simulink model "sampleModel1710"  (R2023a)
settings: Solver=VariableStepAuto  StartTime=0.0  StopTime=10.0  RelTol=1e-3
libraries: hdlsllib x4, simulink x3
settings Model: Creator=user1  LastModifiedBy=user1

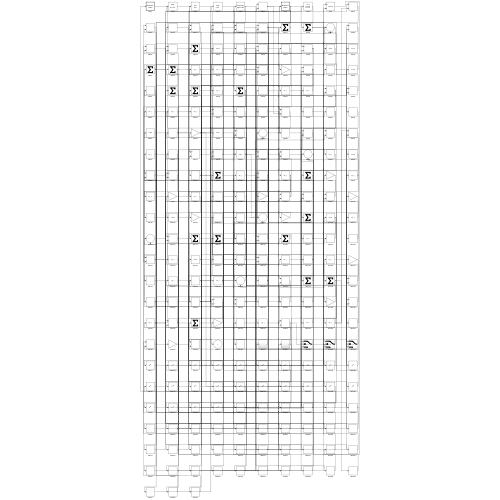
[thumbnail: Simulink's stored preview of the top-level diagram]
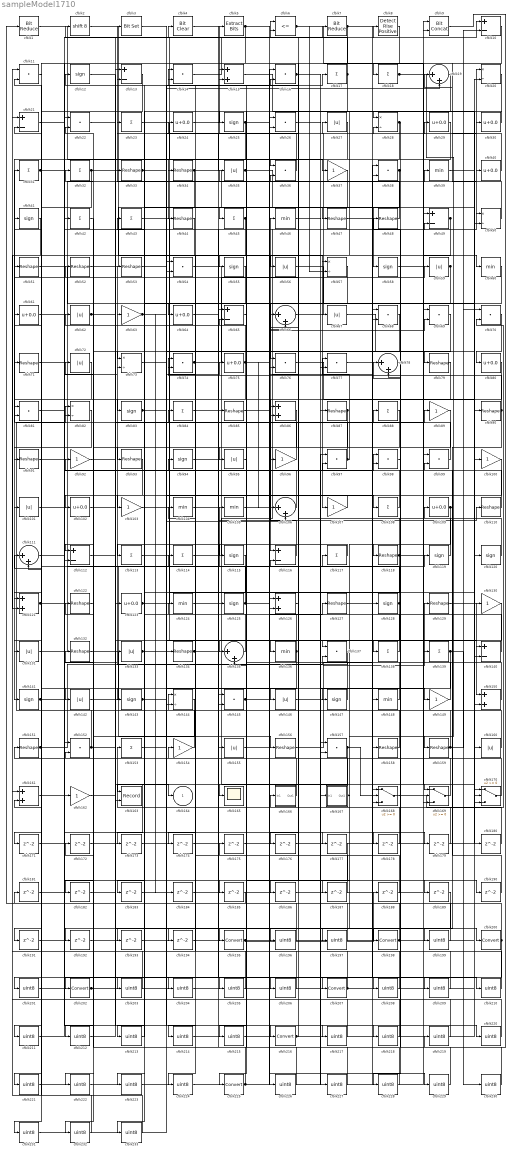
== system sampleModel1710 ==
  cfblk1 : hdlsllib/Logic and Bit Operations/Bit Reduce  mode=AND
  cfblk{10,13,21,49,65,112,116,140} (8 alike) : Sum  Inputs=+-
  cfblk{37,63,89,92,96,100,103,107,130,149,154,162} (12 alike) : Gain
  cfblk{27,35,56,59,62,67,72,95,101,131,133,142,146,155,160} (15 alike) : Abs  SaturateOnIntegerOverflow=off
  cfblk{24,29..30,40,61,64,75,80,102,109,123} (11 alike) : Bias  Bias=0.0  SaturateOnIntegerOverflow=off
  cfblk{39,46,60,104..105,124,136,148} (8 alike) : MinMax
  cfblk{19,66,78,106,111,135} (6 alike) : Sum  Inputs=|++
  cfblk{17..18,23,31..32,42..43,45,84,88,108,113..114,117,138..139,153} (17 alike) : Sum  Inputs=+
  cfblk{11,14,16,22,26,36,38,54,68..70,74,76..77,81,97..99,137,145,152,157} (22 alike) : DotProduct  OutDataTypeStr=Inherit: Inherit via internal rule
  cfblk{33..34,44,47..48,51..53,71,79,85,87,90..91,93,110,118,122,127,129,132,134,151,156,158..159} (26 alike) : Reshape
  cfblk{12,25,41,55,58,83,94,115,119..120,125,128,141,143,147} (15 alike) : Signum
  cfblk{15,86,121,126,150,161} (6 alike) : Sum
  cfblk{20,28,50,57,73,82,144} (7 alike) : Product  Inputs=*/  RndMeth=Zero  SaturateOnIntegerOverflow=on
  cfblk163 : Record  FileSettingsInternal="{\"entries\":[{\"content\":{\"excelSettings\":{\"content\":{},\"type\":\"Streamout.ExcelSettings\"}},\"type\":\"Streamout.FileSettingStorage\",\"uuid\":\"\"}],\"packageUris\":[\"http:\\/\\/schema.mathworks.com\\/mf0\\/streamout_blocks\\/R2020a\"],\"version\":\"1.0\"}"  Layout=[1 1]  SignalsInternal="{\"entries\":[{\"content\":{\"signals\":[{\"content\":{\"blockPath\":[],\"dimensions\":[1],\"domain\":\"\",\"lineColor\":\"#a2142f\",\"plots\":[1],\"port\":1,\"signalID\":3197,\"signalName\":\"XY Graph:1\"},\"type\":\"RecordBlkView.Signal\",\"uuid\":\"\"},{\"content\":{\"blockPath\":[],\"dimensions\":[1],\"domain\":\"\",\"lineColor\":\"#139fff\",\"plots\":[1],\"port\":2,\"signalID\":3200,\"signalName\":\"XY Graph:2\"},\"type\":\"RecordBlkView.Signal\",\"uuid\":\"\"}]},\"type\":\"RecordBlkView.InputSignals\",\"uuid\":\"\"}],\"packageUris\":[\"http:\\/\\/schema.mathworks.com\\/mf0\\/streamout_blocks\\/R2020a\"],\"version\":\"1.0\"}"  VisualizationBindings="{\"xyplotplugin\":{\"info\":[{\"series\":[{\"bindingParametersList\":[{\"parameter\":\"X-Axis\",\"signalID\":3197,\"signalName\":\"XY Graph:1\"},{\"parameter\":\"Y-Axis\",\"signalID\":3200,\"signalName\":\"XY Graph:2\"}],\"seriesID\":41778}],\"subplotID\":1}]}}"  CompatibilityTag=XY  st=-1
  cfblk165 : Scope
  cfblk166 : Subsystem
      settings: LibrarySourceBlock=|
      | hdlsllib/Ports &
      | Subsystems/Subsystem
  cfblk167 : Subsystem
      settings: LibrarySourceBlock=|
      | hdlsllib/Ports &
      | Subsystems/Subsystem
  cfblk168 : Switch  SaturateOnIntegerOverflow=off  InputSameDT=off
  cfblk169 : Switch  SaturateOnIntegerOverflow=off  InputSameDT=off
  cfblk170 : Switch  SaturateOnIntegerOverflow=off  InputSameDT=off
  cfblk{171..194} (24 alike) : Delay  SampleTime=1
  cfblk{195,198,200,202,207,216,225} (7 alike) : DataTypeConversion  SaturateOnIntegerOverflow=off  RndMeth=Floor
  cfblk{196..197,199,201,203..206,208..215,217..224,226..233} (32 alike) : DataTypeConversion  OutDataTypeStr=uint8  SaturateOnIntegerOverflow=off  RndMeth=Floor
  cfblk2 : ArithShift  BitShiftNumber=8
  cfblk3 : simulink/Logic and Bit Operations/Bit Set  iBit=0
      settings: LibrarySourceBlock=|
      | hdlsllib/Logic and Bit
      | Operations/Bit Set
  cfblk4 : simulink/Logic and Bit Operations/Bit Clear  iBit=0
      settings: LibrarySourceBlock=|
      | hdlsllib/Logic and Bit
      | Operations/Bit Clear
  cfblk5 : simulink/Logic and Bit Operations/Extract Bits  bitsToExtract=Upper half  numBits=8  bitIdxRange=[0 7]  outScalingMode=Preserve fixed-point scaling
      settings: LibrarySourceBlock=|
      | hdlsllib/Logic and Bit
      | Operations/Extract Bits
  cfblk6 : RelationalOperator  Operator=<=  OutDataTypeStr=boolean  InputSameDT=off
  cfblk7 : hdlsllib/Logic and Bit Operations/Bit Reduce  mode=AND
  cfblk8 : hdlsllib/Logic and Bit Operations/Detect Rise Positive  vinit=0  OutDataTypeStr=boolean
  cfblk9 : hdlsllib/Logic and Bit Operations/Bit Concat  numInputs=2
  cfblk164 : Outport  VectorParamsAs1DForOutWhenUnconnected=off
  wires:
  cfblk167/1(Out1) -> cfblk154/1, cfblk187/1
  cfblk116/1 -> cfblk46/1
  cfblk131/1 -> cfblk39/1
  cfblk159/1 -> cfblk70/1, cfblk10/2, cfblk76/2
  cfblk154/1 -> cfblk82/1
  cfblk16/1 -> cfblk28/1, cfblk149/1, cfblk176/1
  cfblk82/1 -> cfblk141/1
  cfblk36/1 -> cfblk5/1
  cfblk27/1 -> cfblk101/1
  cfblk43/1 -> cfblk137/1
  cfblk52/1 -> cfblk45/1
  cfblk18/1 -> cfblk153/1, cfblk60/1
  cfblk137/1 -> cfblk53/1
  cfblk80/1 -> cfblk116/1
  cfblk72/1 -> cfblk131/1
  cfblk153/1 -> cfblk134/1
  cfblk123/1 -> cfblk8/1, cfblk33/1
  cfblk158/1 -> cfblk144/1
  cfblk44/1 -> cfblk93/1
  cfblk40/1 -> cfblk18/1
  cfblk108/1 -> cfblk63/1
  cfblk54/1 -> cfblk169/1
  cfblk97/1 -> cfblk32/1, cfblk77/1
  cfblk146/1 -> cfblk129/1
  cfblk170/1 -> cfblk72/1
  cfblk30/1 -> cfblk25/1
  cfblk151/1 -> cfblk137/2, cfblk133/1
  cfblk2/1 -> cfblk107/1
  cfblk168/1 -> cfblk70/2
  cfblk125/1 -> cfblk105/1, cfblk28/2
  cfblk141/1 -> cfblk42/1, cfblk201/1
  cfblk23/1 -> cfblk36/1
  cfblk95/1 -> cfblk165/1
  cfblk88/1 -> cfblk136/1
  cfblk105/1 -> cfblk20/1
  cfblk136/1 -> cfblk14/2, cfblk171/1
  cfblk50/1 -> cfblk19/1
  cfblk66/1 -> cfblk30/1
  cfblk75/1 -> cfblk62/1, cfblk82/2, cfblk106/1, cfblk69/2
  cfblk24/1 -> cfblk67/1
  cfblk74/1 -> cfblk59/1, cfblk14/1
  cfblk51/1 -> cfblk76/1
  cfblk99/1 -> cfblk31/1
  cfblk65/1 -> cfblk225/1
  cfblk109/1 -> cfblk197/1, cfblk199/1
  cfblk48/1 -> cfblk3/1
  cfblk19/1 -> cfblk95/1
  cfblk132/1 -> cfblk156/1
  cfblk32/1 -> cfblk47/1, cfblk81/1
  cfblk104/1 -> cfblk207/1
  cfblk46/1 -> cfblk87/1
  cfblk117/1 -> cfblk113/1
  cfblk37/1 -> cfblk163/1
  cfblk45/1 -> cfblk112/1, cfblk224/1
  cfblk93/1 -> cfblk103/1
  cfblk14/1 -> cfblk6/1
  cfblk90/1 -> cfblk74/1, cfblk159/1
  cfblk126/1 -> cfblk66/1
  cfblk135/1 -> cfblk84/1
  cfblk169/1 -> cfblk94/1
  cfblk70/1 -> cfblk80/1
  cfblk94/1 -> cfblk146/1
  cfblk68/1 -> cfblk142/1
  cfblk160/1 -> cfblk61/1
  cfblk35/1 -> cfblk58/1, cfblk50/2
  cfblk83/1 -> cfblk135/1, cfblk35/1
  cfblk59/1 -> cfblk64/1, cfblk233/1
  cfblk92/1 -> cfblk89/1
  cfblk152/1 -> cfblk111/1, cfblk208/1
  cfblk129/1 -> cfblk150/1
  cfblk157/1 -> cfblk168/2, cfblk173/1
  cfblk25/1 -> cfblk44/1, cfblk37/1
  cfblk87/1 -> cfblk96/1, cfblk174/1
  cfblk5/1 -> cfblk91/1, cfblk229/1
  cfblk15/1 -> cfblk160/1
  cfblk111/1 -> cfblk98/1
  cfblk1/1 -> cfblk34/1
  cfblk106/1 -> cfblk52/1
  cfblk134/1 -> cfblk50/1, cfblk110/1
  cfblk28/1 -> cfblk138/1, cfblk183/1
  cfblk166/1(Out1) -> cfblk41/1
  cfblk112/1 -> cfblk164/1
  cfblk63/1 -> cfblk27/1, cfblk184/1, cfblk220/1
  cfblk53/1 -> cfblk17/1
  cfblk138/1 -> cfblk43/1
  cfblk33/1 -> cfblk77/2, cfblk193/1
  cfblk79/1 -> cfblk135/2
  cfblk110/1 -> cfblk36/2
  cfblk7/1 -> cfblk158/1, cfblk111/2, cfblk144/2
  cfblk150/1 -> cfblk88/1
  cfblk121/1 -> cfblk85/1, cfblk73/2
  cfblk73/1 -> cfblk19/2
  cfblk29/1 -> cfblk121/1
  cfblk6/1 -> cfblk139/1, cfblk57/2
  cfblk107/1 -> cfblk102/1
  cfblk67/1 -> cfblk120/1
  cfblk148/1 -> cfblk92/1
  cfblk77/1 -> cfblk148/1
  cfblk120/1 -> cfblk51/1
  cfblk34/1 -> cfblk126/1, cfblk73/1, cfblk29/1
  cfblk142/1 -> cfblk26/2
  cfblk49/1 -> cfblk55/1, cfblk191/1
  cfblk55/1 -> cfblk143/1
  cfblk8/1 -> cfblk112/2
  cfblk145/1 -> cfblk127/1, cfblk97/2
  cfblk155/1 -> cfblk200/1
  cfblk71/1 -> cfblk49/2
  cfblk103/1 -> cfblk145/2
  cfblk76/1 -> cfblk130/1
  cfblk113/1 -> cfblk170/1
  cfblk62/1 -> cfblk4/1, cfblk190/1
  cfblk140/1 -> cfblk114/1
  cfblk4/1 -> cfblk125/1
  cfblk41/1 -> cfblk121/2
  cfblk98/1 -> cfblk48/1
  cfblk58/1 -> cfblk140/1
  cfblk149/1 -> cfblk15/1
  cfblk119/1 -> cfblk109/1
  cfblk60/1 -> cfblk118/1
  cfblk61/1 -> cfblk162/1
  cfblk124/1 -> cfblk198/1
  cfblk139/1 -> cfblk157/2, cfblk230/1
  cfblk84/1 -> cfblk140/2
  cfblk38/1 -> cfblk115/1, cfblk203/1
  cfblk128/1 -> cfblk81/2, cfblk213/1
  cfblk20/1 -> cfblk57/1
  cfblk114/1 -> cfblk40/1
  cfblk96/1 -> cfblk71/1
  cfblk122/1 -> cfblk202/1
  cfblk22/1 -> cfblk195/1
  cfblk161/1 -> cfblk216/1
  cfblk81/1 -> cfblk10/1
  cfblk130/1 -> cfblk163/2
  cfblk133/1 -> cfblk117/1, cfblk106/2
  cfblk17/1 -> cfblk2/1, cfblk83/1
  cfblk118/1 -> cfblk15/2, cfblk23/1, cfblk170/3, cfblk223/1
  cfblk127/1 -> cfblk68/2
  cfblk3/1 -> cfblk108/1
  cfblk64/1 -> cfblk79/1
  cfblk143/1 -> cfblk119/1, cfblk147/1, cfblk75/1
  cfblk147/1 -> cfblk12/1
  cfblk10/1 -> cfblk56/1
  cfblk56/1 -> cfblk170/2
  cfblk31/1 -> cfblk7/1, cfblk206/1
  cfblk156/1 -> cfblk38/1
  cfblk171/1 -> cfblk169/2
  cfblk172/1 -> cfblk54/2
  cfblk173/1 -> cfblk26/1
  cfblk174/1 -> cfblk150/2
  cfblk175/1 -> cfblk168/1
  cfblk176/1 -> cfblk49/1
  cfblk102/1 -> cfblk177/1
  cfblk91/1 -> cfblk178/1
  cfblk178/1 -> cfblk145/1
  cfblk162/1 -> cfblk179/1
  cfblk179/1 -> cfblk116/2
  cfblk39/1 -> cfblk180/1
  cfblk180/1 -> cfblk6/2
  cfblk89/1 -> cfblk182/1
  cfblk183/1 -> cfblk168/3
  cfblk184/1 -> cfblk169/3
  cfblk101/1 -> cfblk185/1
  cfblk185/1 -> cfblk1/1
  cfblk69/1 -> cfblk186/1
  cfblk187/1 -> cfblk74/2
  cfblk188/1 -> cfblk157/1
  cfblk12/1 -> cfblk189/1
  cfblk190/1 -> cfblk99/2
  cfblk191/1 -> cfblk38/2
  cfblk144/1 -> cfblk192/1
  cfblk192/1 -> cfblk68/1
  cfblk193/1 -> cfblk66/2
  cfblk115/1 -> cfblk194/1
  cfblk194/1 -> cfblk126/2
  cfblk195/1 -> cfblk188/1, cfblk175/1, cfblk20/2
  cfblk196/1 -> cfblk22/1
  cfblk197/1 -> cfblk22/2
  cfblk198/1 -> cfblk196/1, cfblk151/1
  cfblk199/1 -> cfblk124/1
  cfblk200/1 -> cfblk69/1, cfblk221/1
  cfblk201/1 -> cfblk155/1
  cfblk202/1 -> cfblk123/1, cfblk99/1
  cfblk203/1 -> cfblk122/1
  cfblk21/1 -> cfblk204/1
  cfblk204/1 -> cfblk90/1
  cfblk177/1 -> cfblk205/1
  cfblk205/1 -> cfblk21/1
  cfblk206/1 -> cfblk21/2
  cfblk207/1 -> cfblk16/2, cfblk24/1
  cfblk208/1 -> cfblk104/1
  cfblk181/1 -> cfblk209/1
  cfblk209/1 -> cfblk152/2
  cfblk47/1 -> cfblk210/1
  cfblk210/1 -> cfblk181/1
  cfblk13/1 -> cfblk211/1
  cfblk211/1 -> cfblk152/1
  cfblk42/1 -> cfblk212/1
  cfblk212/1 -> cfblk13/1
  cfblk213/1 -> cfblk13/2
  cfblk100/1 -> cfblk214/1
  cfblk214/1 -> cfblk167/1(In1)
  cfblk57/1 -> cfblk215/1
  cfblk215/1 -> cfblk100/1
  cfblk216/1 -> cfblk98/2, cfblk166/1(In1)
  cfblk182/1 -> cfblk217/1
  cfblk217/1 -> cfblk161/1
  cfblk26/1 -> cfblk218/1
  cfblk218/1 -> cfblk161/2
  cfblk9/1 -> cfblk219/1
  cfblk219/1 -> cfblk16/1
  cfblk220/1 -> cfblk9/1
  cfblk221/1 -> cfblk9/2
  cfblk86/1 -> cfblk222/1
  cfblk222/1 -> cfblk97/1
  cfblk223/1 -> cfblk86/1
  cfblk224/1 -> cfblk86/2
  cfblk225/1 -> cfblk128/1, cfblk132/1
  cfblk85/1 -> cfblk226/1
  cfblk226/1 -> cfblk65/1
  cfblk186/1 -> cfblk227/1
  cfblk227/1 -> cfblk65/2
  cfblk78/1 -> cfblk228/1
  cfblk228/1 -> cfblk172/1
  cfblk229/1 -> cfblk78/1
  cfblk230/1 -> cfblk78/2
  cfblk11/1 -> cfblk231/1
  cfblk231/1 -> cfblk54/1
  cfblk189/1 -> cfblk232/1
  cfblk232/1 -> cfblk11/1
  cfblk233/1 -> cfblk11/2

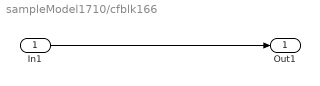
== system sampleModel1710/cfblk166 ==
  In1 : Inport
  Out1 : Outport
  wires:
  In1/1 -> Out1/1

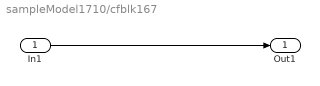
== system sampleModel1710/cfblk167 ==
  In1 : Inport
  Out1 : Outport
  wires:
  In1/1 -> Out1/1
